simulink model "Differential_Jacobian_mapping_Model"  (R2016a)
settings: Solver=FixedStepAuto  SolverMode=SingleTasking  StartTime=0  StopTime=2  FixedStep=0.04  RelTol=1e-3
undefined symbols (not defined in the file): display, Z
libraries: sm_lib x176, nesl_utility x21, simulink x10
(part 1 of 2)
settings Model: Creator=Andrew  LastModifiedBy=wul20

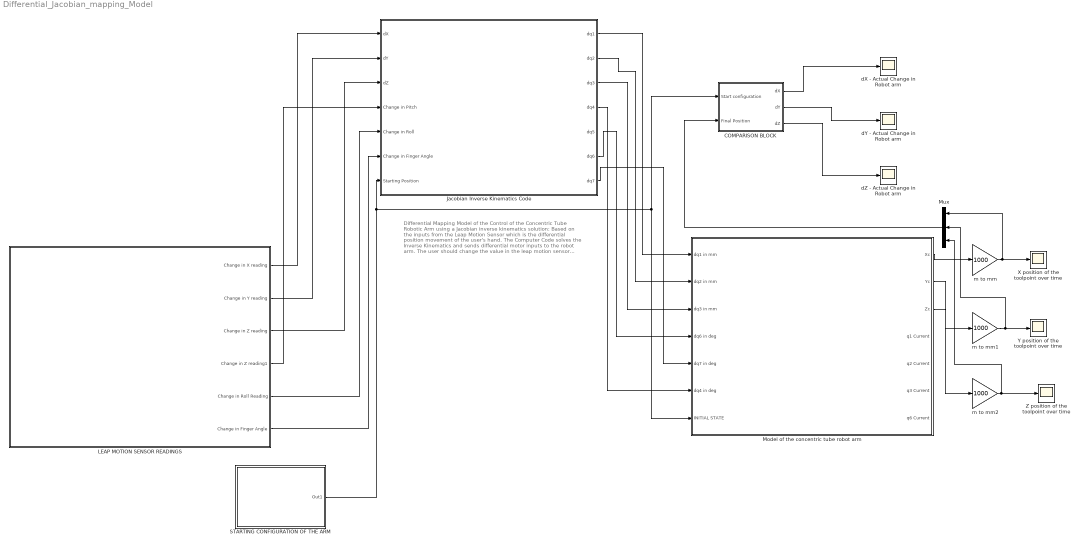
== system Differential_Jacobian_mapping_Model ==
  note: Differential Mapping Model of the Control of
      | the Concentric Tube Robotic Arm using a Jacobian inverse kinematics solution:
      |
      | Based on the inputs from the Leap Motion Sensor which is the differential position movement of the user's hand.
      | The Computer Code solves the Inverse Kinematics and sends differential motor inputs to the robot arm.
      |
      | The user should change the value in the leap motion sensor readings and see how the differential mapping model sends the right motor commands to the arm for it to reach the desired position-change recorded in the scopes from the comparison block.
      |
      | The extrusion takes about 1 simulation second in this simulation every time it elongates to its target position
  COMPARISON BLOCK : Subsystem
  Jacobian Inverse Kinematics Code : Subsystem
      mask Display: image('computer.png');
  LEAP MOTION SENSOR READINGS : Subsystem  mask{X=10, Y=-10, Z=10, P=0, R=90, d=60}
      mask prompts: X "Change in Toolpoint X position (mm)"; Y "Change in Toolpoint Y position (mm)"; Z "Change in Toolpoint Z position (mm)"; P "Change in hand pitch position (degrees)"; R "Change in Roll Angle (degrees)"; d "Change in Finger angle (degrees)"
      mask help: Write down the target differential displacement and orientation:
      mask Display: image('Leap motion Sensor.png');
  Model of the concentric tube robot arm : Subsystem  mask(3D Model of the Concentric Tube Robot Arm){r=173.58}
      mask prompts: r "Radius of curvature in mm"
      mask help:
      | This is a simmechanics model of the robot arm extruding from the origin to its destination in a constant 1 second.
      | Due to the limitations in the model, the maximum extrusion are:
      | tube 1 extrudes a maximum of 100mm (relative)
      | tube 2 extrudes a maximum of 272.67mm that is 90 degrees of curvature (relative)
      | tube 3 extrudes a maximum of 300mm (relative)
      mask init:
      | %set_param('Differential_Jacobian_mapping_Model','AlgebraicLoopSolver','LineSearch')
      | set_param('Differential_Jacobian_mapping_Model','AlgebraicLoopSolver','TrustRegion')
      | 
      | % Geometry 
      | r = 173.58;
      | 
      | %initial Joint conditions:
      | q1 = 10;
      | q2 = 30;
      | q3 = 7;
      | 
      | %Cross section of the Curved Tube
      | x = [-1:0.01:1];
      | y = [sqrt(1-x.^2) -sqrt(1-x.^2)];
      | x = r + x;
      | X = [x'; flip(x)'];
      | Y = y';
      | Cross_section_tube2 = [X, flip(Y)];
      | Cross_section_tube2(202,:)=[];
      | Cross_section_tube2(401,:)=[];
      mask Display: image('Concentric tube robot picture.png');
  Mux : Mux  Inputs=3
  STARTING CONFIGURATION OF THE ARM : Subsystem  mask{q1_in=50, q2_in=50, q3_in=50, q6_in=90, q7_in=0}
      mask prompts: q1_in "Initial q1 elongation (mm)"; q2_in "Initial q2 elongation (mm)"; q3_in "Initial q3 elongation (mm)"; q6_in "Initial q6 rotation (degrees) e.g. 0 degrees means the arm points downwards"; q7_in "Initial q7 rotation (degrees)"
  X position of the toolpoint over time : Scope
  Y position of the toolpoint over time : Scope
  Z position of the toolpoint over time : Scope
  dX - Actual Change in Robot arm : Scope
  dY - Actual Change in Robot arm : Scope
  dZ - Actual Change in Robot arm : Scope
  m to mm : Gain  Gain=1000
  m to mm1 : Gain  Gain=1000
  m to mm2 : Gain  Gain=1000
  wires:
  Model of the concentric tube robot arm/2(Yc) -> m to mm1/1
  Model of the concentric tube robot arm/1(Xc) -> m to mm/1
  Model of the concentric tube robot arm/3(Zc) -> m to mm2/1
  LEAP MOTION SENSOR READINGS/1(Change in X reading) -> Jacobian Inverse Kinematics Code/1(dX)
  LEAP MOTION SENSOR READINGS/2(Change in Y reading) -> Jacobian Inverse Kinematics Code/2(dY)
  LEAP MOTION SENSOR READINGS/3(Change in Z reading) -> Jacobian Inverse Kinematics Code/3(dZ)
  LEAP MOTION SENSOR READINGS/5(Change in Roll Reading) -> Jacobian Inverse Kinematics Code/5(Change in Roll)
  m to mm/1 -> Mux/1, X position of the toolpoint over time/1
  m to mm1/1 -> Mux/2, Y position of the toolpoint over time/1
  m to mm2/1 -> Z position of the toolpoint over time/1, Mux/3
  LEAP MOTION SENSOR READINGS/6(Change in Finger Angle) -> Jacobian Inverse Kinematics Code/6(Change in Finger Angle)
  Jacobian Inverse Kinematics Code/1(dq1) -> Model of the concentric tube robot arm/1(dq1 in mm)
  Jacobian Inverse Kinematics Code/2(dq2) -> Model of the concentric tube robot arm/2(dq2 in mm)
  Jacobian Inverse Kinematics Code/3(dq3) -> Model of the concentric tube robot arm/3(dq3 in mm)
  Jacobian Inverse Kinematics Code/7(dq7) -> Model of the concentric tube robot arm/5(dq7 in deg)
  STARTING CONFIGURATION OF THE ARM/1(Out1) -> Jacobian Inverse Kinematics Code/7(Starting Position), COMPARISON BLOCK/1(Start configuration), Model of the concentric tube robot arm/7(INITIAL STATE)
  Jacobian Inverse Kinematics Code/4(dq4) -> Model of the concentric tube robot arm/6(dq4 in deg)
  Mux/1 -> COMPARISON BLOCK/2(Final Position)
  COMPARISON BLOCK/1(dX) -> dX - Actual Change in Robot arm/1
  COMPARISON BLOCK/2(dY) -> dY - Actual Change in Robot arm/1
  COMPARISON BLOCK/3(dZ) -> dZ - Actual Change in Robot arm/1
  Jacobian Inverse Kinematics Code/6(dq6) -> Model of the concentric tube robot arm/4(dq6 in deg)
  LEAP MOTION SENSOR READINGS/4(Change in Z reading1) -> Jacobian Inverse Kinematics Code/4(Change in Pitch)

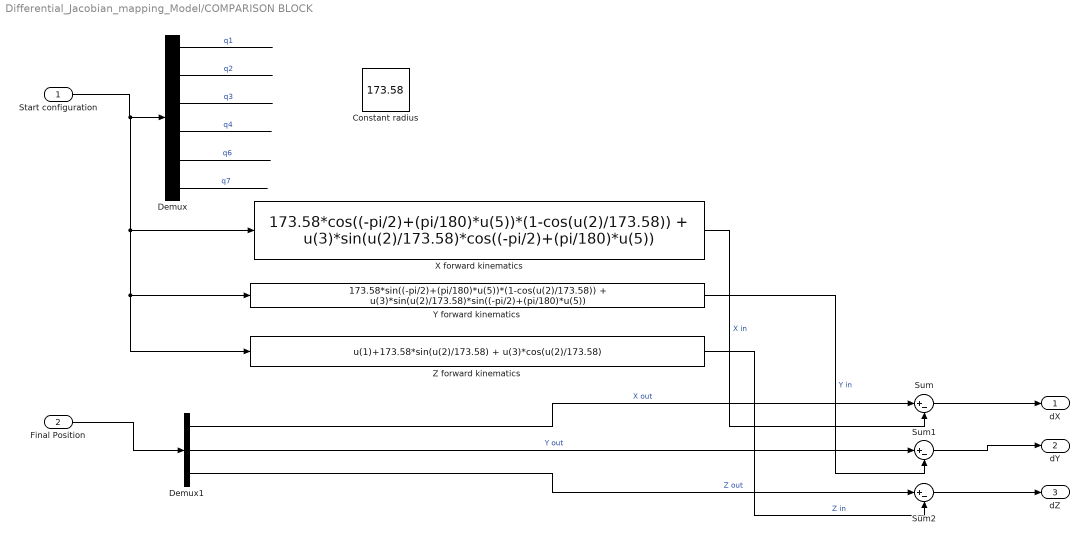
== system Differential_Jacobian_mapping_Model/COMPARISON BLOCK ==
  Start configuration : Inport
  Final Position : Inport  Port=2
  Constant radius : Constant  Value=173.58
  Demux : Demux  Outputs=6
  Demux1 : Demux  Outputs=3
  Sum : Sum  Inputs=|+-
  Sum1 : Sum  Inputs=|+-
  Sum2 : Sum  Inputs=|+-
  X forward kinematics : Fcn  Expr=173.58*cos((-pi/2)+(pi/180)*u(5))*(1-cos(u(2)/173.58)) + u(3)*sin(u(2)/173.58)*cos((-pi/2)+(pi/180)*u(5))
  Y forward kinematics : Fcn  Expr=173.58*sin((-pi/2)+(pi/180)*u(5))*(1-cos(u(2)/173.58)) + u(3)*sin(u(2)/173.58)*sin((-pi/2)+(pi/180)*u(5))
  Z forward kinematics : Fcn  Expr=u(1)+173.58*sin(u(2)/173.58) + u(3)*cos(u(2)/173.58)
  dX : Outport
  dY : Outport  Port=2
  dZ : Outport  Port=3
  wires:
  Start configuration/1 -> Z forward kinematics/1, Y forward kinematics/1, X forward kinematics/1, Demux/1
  Demux/1 -> ?  "q1"
  Demux/2 -> ?  "q2"
  Demux/3 -> ?  "q3"
  Demux/4 -> ?  "q4"
  Demux/5 -> ?  "q6"
  Demux/6 -> ?  "q7"
  X forward kinematics/1 -> Sum/2  "X in"
  Y forward kinematics/1 -> Sum1/2  "Y in"
  Z forward kinematics/1 -> Sum2/2  "Z in"
  Final Position/1 -> Demux1/1
  Demux1/1 -> Sum/1  "X out"
  Demux1/2 -> Sum1/1  "Y out"
  Demux1/3 -> Sum2/1  "Z out"
  Sum2/1 -> dZ/1
  Sum1/1 -> dY/1
  Sum/1 -> dX/1

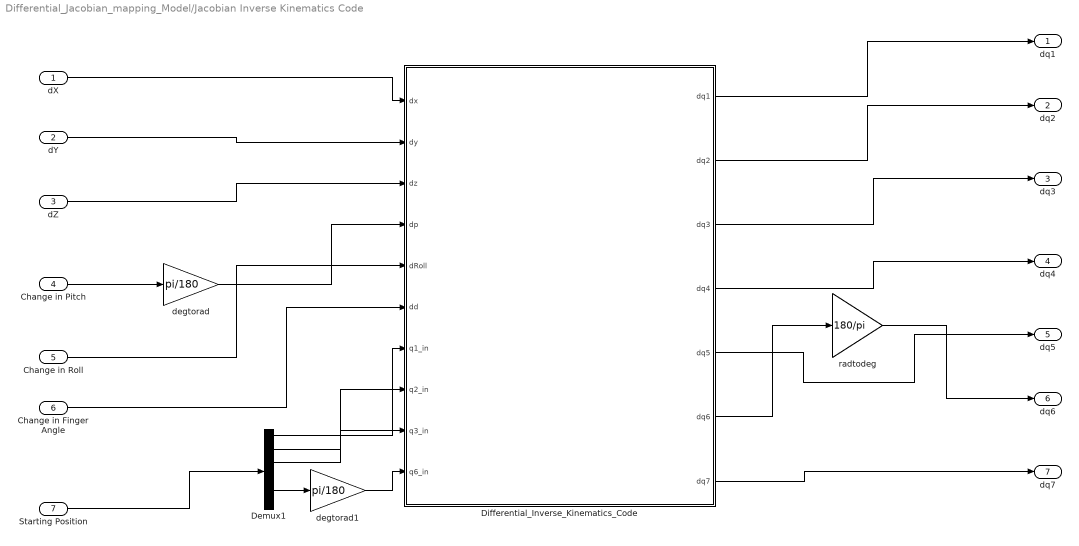
== system Differential_Jacobian_mapping_Model/Jacobian Inverse Kinematics Code ==
  dX : Inport
  dY : Inport  Port=2
  dZ : Inport  Port=3
  Change in Pitch : Inport  Port=4
  Change in Roll : Inport  Port=5
  Change in Finger Angle : Inport  Port=6
  Starting Position : Inport  Port=7
  Demux1 : Demux  Outputs=6
  Differential_Inverse_Kinematics_Code : MATLAB Function  TreatAsAtomicUnit=on
  degtorad : Gain  Gain=pi/180
  degtorad1 : Gain  Gain=pi/180
  radtodeg : Gain  Gain=180/pi
  dq1 : Outport
  dq2 : Outport  Port=2
  dq3 : Outport  Port=3
  dq4 : Outport  Port=4
  dq5 : Outport  Port=5
  dq6 : Outport  Port=6
  dq7 : Outport  Port=7
  wires:
  dX/1 -> Differential_Inverse_Kinematics_Code/1(dx)
  dY/1 -> Differential_Inverse_Kinematics_Code/2(dy)
  dZ/1 -> Differential_Inverse_Kinematics_Code/3(dz)
  Change in Roll/1 -> Differential_Inverse_Kinematics_Code/5(dRoll)
  Differential_Inverse_Kinematics_Code/1(dq1) -> dq1/1
  Differential_Inverse_Kinematics_Code/2(dq2) -> dq2/1
  Differential_Inverse_Kinematics_Code/3(dq3) -> dq3/1
  Differential_Inverse_Kinematics_Code/4(dq4) -> dq4/1
  Differential_Inverse_Kinematics_Code/5(dq5) -> dq5/1
  Differential_Inverse_Kinematics_Code/7(dq7) -> dq7/1
  Change in Pitch/1 -> degtorad/1
  degtorad/1 -> Differential_Inverse_Kinematics_Code/4(dp)
  Differential_Inverse_Kinematics_Code/6(dq6) -> radtodeg/1
  radtodeg/1 -> dq6/1
  Change in Finger Angle/1 -> Differential_Inverse_Kinematics_Code/6(dd)
  Starting Position/1 -> Demux1/1
  Demux1/1 -> Differential_Inverse_Kinematics_Code/7(q1_in)
  Demux1/2 -> Differential_Inverse_Kinematics_Code/8(q2_in)
  Demux1/3 -> Differential_Inverse_Kinematics_Code/9(q3_in)
  degtorad1/1 -> Differential_Inverse_Kinematics_Code/10(q6_in)
  Demux1/5 -> degtorad1/1

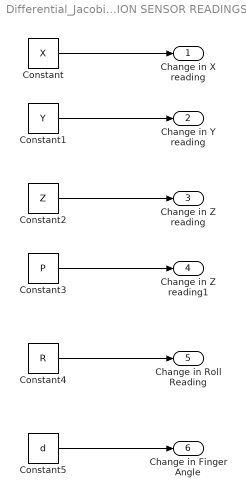
== system Differential_Jacobian_mapping_Model/LEAP MOTION SENSOR READINGS ==
  Constant : Constant  Value=X
  Constant1 : Constant  Value=Y
  Constant2 : Constant  Value=Z
  Constant3 : Constant  Value=P
  Constant4 : Constant  Value=R
  Constant5 : Constant  Value=d
  Change in X reading : Outport
  Change in Y reading : Outport  Port=2
  Change in Z reading : Outport  Port=3
  Change in Z reading1 : Outport  Port=4
  Change in Roll Reading : Outport  Port=5
  Change in Finger Angle : Outport  Port=6
  wires:
  Constant/1 -> Change in X reading/1
  Constant1/1 -> Change in Y reading/1
  Constant2/1 -> Change in Z reading/1
  Constant4/1 -> Change in Roll Reading/1
  Constant5/1 -> Change in Finger Angle/1
  Constant3/1 -> Change in Z reading1/1

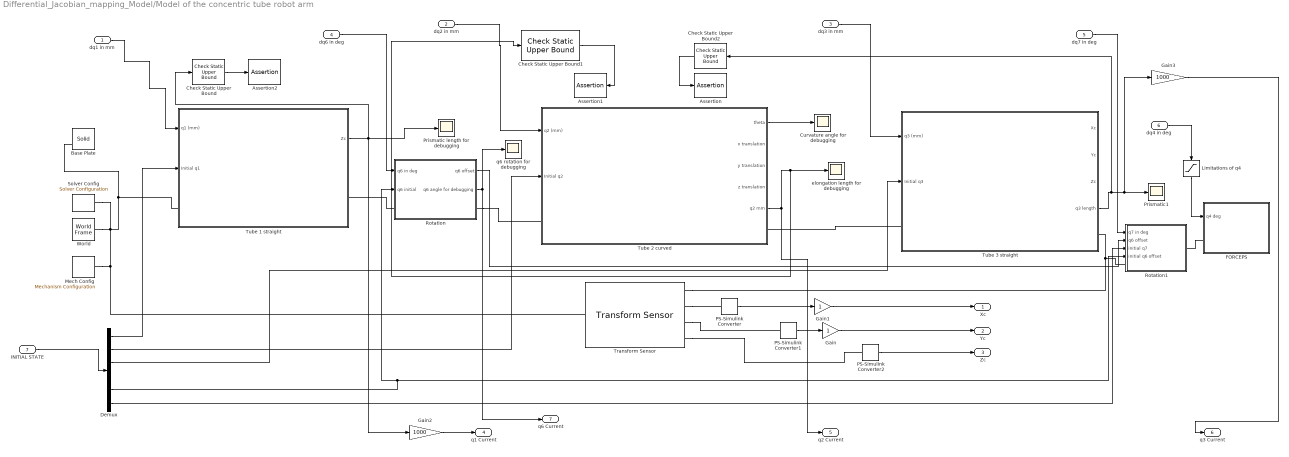
== system Differential_Jacobian_mapping_Model/Model of the concentric tube robot arm ==
  dq1 in mm : Inport
  dq2 in mm : Inport  Port=2
  dq3 in mm : Inport  Port=3
  dq6 in deg : Inport  Port=4
  dq7 in deg : Inport  Port=5
  dq4 in deg : Inport  Port=6
  INITIAL STATE : Inport  Port=7
  Assertion : Assertion  AssertionFailFcn=display('Warning: Tube 3 has reached maximum elongation. You may get an inaccurate position')  StopWhenAssertionFail=off
  Assertion1 : Assertion  AssertionFailFcn=display('Warning: Tube 2 has reached maximum elongation. You may get an inaccurate position')  StopWhenAssertionFail=off
  Assertion2 : Assertion  AssertionFailFcn=display('Warning: Tube 1 has reached maximum elongation. You may get an inaccurate position')  StopWhenAssertionFail=off
  Base Plate : sm_lib/Body Elements/Solid  InertiaType=CalculateFromGeometry  Mass=1  MassUnits=kg  CenterOfMass=[0 0 0]  CenterOfMassUnits=m  MomentsOfInertia=[1 1 1]  MomentsOfInertiaUnits=kg*m^2  ProductsOfInertia=[0 0 0]  ProductsOfInertiaUnits=kg*m^2  DensityBased=on  Density=1000  DensityUnits=kg/(m^3)  DoExposeReferenceFrame=on  SerializedFrames=<Frames><Frame><Id>Frame1</Id><Value><Name>B</Name><Origin><Source>GeometricFeature</Source><FeatureName>+z surface</FeatureName></Origin><PrimaryAxis><DefinedDirection>+Z</DefinedDirection><Source>ReferenceFrame</Source><SourceDirection>+Z</SourceDirection><FeatureName></FeatureName></PrimaryAxis><SecondaryAxis><DefinedDirection>+X</DefinedDirection><Source>ReferenceFrame</Source><SourceDirection>+X</SourceDirection><FeatureName></FeatureName></SecondaryAxis></Value></Frame><Frame><Id>Frame2</Id><Value><Name>F2</Name><Origin><Source>GeometricFeature</Source><FeatureName>+z surface</FeatureName></Origin><PrimaryAxis><DefinedDirection>+Z</DefinedDirection><Source>ReferenceFrame</Source><SourceDirection>+Z</SourceDirection><FeatureName></FeatureName></PrimaryAxis><SecondaryAxis><DefinedDirection>+X</DefinedDirection><Source>ReferenceFrame</Source><SourceDirection>+X</SourceDirection><FeatureName></FeatureName></SecondaryAxis></Value></Frame></Frames>  GraphicType=FromGeometry  MarkerShape=Sphere  MarkerSize=10  GraphicVisPropType=SimpleVisualProperties  GraphicDiffuseColor=[0.4 0.4 0.4]  GraphicSpecularColor=[0.5 0.5 0.5 1.0]  GraphicAmbientColor=[0.15 0.15 0.15 1.0]  GraphicEmissiveColor=[0.0 0.0 0.0 1.0]  GraphicShininess=75  GraphicOpacity=1.0  GeometryShape=Brick  RectangleSize=[1 1]  RectangleSizeUnits=m  BrickDimensions=[100 100 500]  BrickDimensionUnits=mm  CylinderRadius=1  CylinderRadiusUnits=m  CylinderLength=1  CylinderLengthUnits=m  SphereRadius=1  SphereRadiusUnits=m  EllipsoidRadii=[1 1 1]  EllipsoidRadiiUnits=m  ExtrusionCrossSection=10  ExtrusionCrossSectionUnits=cm  ExtrusionLength=10  ExtrusionLengthUnits=cm  PolygonNumSides=3  PolygonOuterRadius=1  PolygonOuterRadiusUnits=m  ExtGeomFileType=STL  ExtGeomFileUnits=m  RevolutionCrossSection=[1 1; 1 -1; 2 -1; 2 1]  RevolutionCrossSectionUnits=m  RevolutionExtent=Full  RevolutionAngle=180  RevolutionAngleUnits=deg
  Check Static Upper Bound : simulink/Model Verification/Check Static  Upper Bound  Description=u <= 0.07725  max=0.07725  max_included=on  enabled=off  callback=Warning: Tube 1 has reached maximum elongation. You may get inaccurate position  stopWhenAssertionFail=off  export=on  icon=text
  Check Static Upper Bound1 : simulink/Model Verification/Check Static  Upper Bound  Description=u <= 82.5  max=82.5  max_included=on  enabled=off  callback=Warning: Tube 2 has reached maximum elongation. You may get inaccurate position  stopWhenAssertionFail=off  export=on  icon=graphic
  Check Static Upper Bound2 : simulink/Model Verification/Check Static  Upper Bound  Description=u <= 0.0975  max=0.0975  max_included=on  enabled=off  callback="\"Warning: Tube 3 has reached maximum elongation. You may get an inaccurate position\""  stopWhenAssertionFail=off  export=on  icon=text
      settings: AttributesFormatString=%<callback>
  Curvature angle for debugging : Scope
  Demux : Demux  Outputs=6
  FORCEPS : Subsystem
      mask Display: image('Forceps.png');
  Gain : Gain
  Gain1 : Gain
  Gain2 : Gain  Gain=1000
  Gain3 : Gain  Gain=1000
  Limitations of q4 : Saturate  UpperLimit=60  LowerLimit=0
  Mech Config : sm_lib/Utilities/Mechanism Configuration  UniformGravity=Constant  GravityVector=[0 0 -9.80665]  GravityUnits=m/s^2  LinearizationDelta=0.001
  PS-Simulink Converter : nesl_utility/PS-Simulink Converter  PhysicalDomain=network_engine_domain  SubClassName=ps_output  LeftPortType=input  RightPortType=output  PseudoPeriodic=off  Frequencies=[]  Unit=1  AffineConversion=off
  PS-Simulink Converter1 : nesl_utility/PS-Simulink Converter  PhysicalDomain=network_engine_domain  SubClassName=ps_output  LeftPortType=input  RightPortType=output  PseudoPeriodic=off  Frequencies=[]  Unit=1  AffineConversion=off
  PS-Simulink Converter2 : nesl_utility/PS-Simulink Converter  PhysicalDomain=network_engine_domain  SubClassName=ps_output  LeftPortType=input  RightPortType=output  PseudoPeriodic=off  Frequencies=[]  Unit=1  AffineConversion=off
  Prismatic length for debugging : Scope
  Prismatic1 : Scope
  Rotation : Subsystem
  Rotation1 : Subsystem
  Solver Config : nesl_utility/Solver Configuration  PhysicalDomain=network_engine_domain  SubClassName=solver  LeftPortType=input  RightPortType=generic  Accelerate=off  Tones=[]  Harmonics=[]  SimulateNoise=off  Profile=off  UseLocalSampling=off  EnableSwitchedLinearOptims=on  FrequencyDomain=off  UseCCode=off  RelTol=0.001  AbsTol=1e-06  MinStep=1e-09  ToWorkspace=off  RevertToSquareIcSolve=off  NumHomotopyIterations=100  PhasorMode=off  PhasorModeNumHarmonics=1  OverrideAbsTol=off  DoDC=off  ResidualTolerance=1e-06  UseLocalSolver=off  LocalSolverChoice=NE_BACKWARD_EULER_ADVANCER  LocalSolverSampleTime=0.001  DoFixedCost=off  MaxNonlinIter=3  MaxModeIter=2  LinearAlgebra=Sparse  DelaysMemoryBudget=1024  AutomaticFiltering=on  FilteringTimeConstant=0.001
  Transform Sensor : sm_lib/Frames and Transforms/Transform Sensor  MeasurementFrame=Base  SenseAngle=off  SenseAxis=off  SenseAngle1=off  SenseAngle2=off  SenseAngle3=off  SenseQ=off  SenseR=off  SenseOmegaX=off  SenseOmegaY=off  SenseOmegaZ=off  SenseOmega1=off  SenseOmega2=off  SenseOmega3=off  SenseQDot=off  SenseRDot=off  SenseAlphaX=off  SenseAlphaY=off  SenseAlphaZ=off  SenseAlpha1=off  SenseAlpha2=off  SenseAlpha3=off  SenseQDDot=off  SenseRDDot=off  SenseX=on  SenseY=on  SenseZ=on  SenseRad=off  SenseAzim=off  SenseDist=off  SenseInc=off  SenseXDot=off  SenseYDot=off  SenseZDot=off  SenseRadDot=off  SenseAzimDot=off  SenseDistDot=off  SenseIncDot=off  SenseXDDot=off  SenseYDDot=off  SenseZDDot=off  SenseRadDDot=off  SenseAzimDDot=off  SenseDistDDot=off  SenseIncDDot=off
  Tube 1 straight : Subsystem
      mask Display: image('straight tube.png');
  Tube 2 curved : Subsystem
      mask Display: image('The curved tube.png');
  Tube 3 straight : Subsystem
      mask Display: image('straight tube.png');
  World : sm_lib/Frames and Transforms/World Frame
  elongation length for debugging : Scope
  q6 rotation for debugging : Scope
  Xc : Outport
  Yc : Outport  Port=2
  Zc : Outport  Port=3
  q1 Current : Outport  Port=4
  q2 Current : Outport  Port=5
  q3 Current : Outport  Port=6
  q6 Current : Outport  Port=7
  wires:
  dq1 in mm/1 -> Tube 1 straight/1(q1 (mm))
  dq2 in mm/1 -> Tube 2 curved/1(q2 (mm))
  dq3 in mm/1 -> Tube 3 straight/1(q3 (mm))
  PS-Simulink Converter1/1 -> Gain/1
  PS-Simulink Converter2/1 -> Zc/1
  PS-Simulink Converter/1 -> Gain1/1
  Gain/1 -> Yc/1
  dq6 in deg/1 -> Rotation/1(q6 in deg)
  dq7 in deg/1 -> Rotation1/1(q7 in deg)
  dq4 in deg/1 -> Limitations of q4/1
  Limitations of q4/1 -> FORCEPS/1(q4 deg)
  Tube 1 straight/1(Zc) -> Gain2/1, Check Static Upper Bound/1, Prismatic length for debugging/1
  Tube 2 curved/1(theta) -> Curvature angle for debugging/1
  Rotation/1(q6 offset) -> Rotation1/2(q6 offset)
  Check Static Upper Bound2/1 -> Assertion/1
  Check Static Upper Bound1/1 -> Assertion1/1
  Check Static Upper Bound/1 -> Assertion2/1
  Gain1/1 -> Xc/1
  INITIAL STATE/1 -> Demux/1
  Demux/1 -> Tube 1 straight/2(Initial q1)
  Demux/5 -> Rotation1/4(initial q6 offset), Rotation/2(q6 initial)
  Demux/2 -> Tube 2 curved/2(Initial q2)
  Demux/3 -> Tube 3 straight/2(Initial q3)
  Demux/6 -> Rotation1/3(initial q7)
  Rotation/2(q6 angle for debugging) -> q6 rotation for debugging/1, q6 Current/1
  Tube 3 straight/4(q3 length) -> Check Static Upper Bound2/1, Gain3/1, Prismatic1/1
  Tube 2 curved/5(q2 mm) -> Check Static Upper Bound1/1, elongation length for debugging/1, q2 Current/1
  Gain2/1 -> q1 Current/1
  Gain3/1 -> q3 Current/1
  connections:
  World/RConn1 -- Transform Sensor/LConn1 -- Mech Config/RConn1 -- Tube 1 straight/LConn1 -- Base Plate/LConn2 -- Solver Config/RConn1
  Tube 3 straight/LConn1 -- Tube 2 curved/RConn1
  Transform Sensor/RConn4 -- PS-Simulink Converter2/LConn1
  Transform Sensor/RConn1 -- Tube 3 straight/RConn1 -- Rotation1/LConn1
  Rotation/LConn1 -- Tube 1 straight/RConn1
  Rotation/RConn1 -- Tube 2 curved/LConn1
  FORCEPS/LConn1 -- Rotation1/RConn1
  Transform Sensor/RConn3 -- PS-Simulink Converter1/LConn1
  Transform Sensor/RConn2 -- PS-Simulink Converter/LConn1

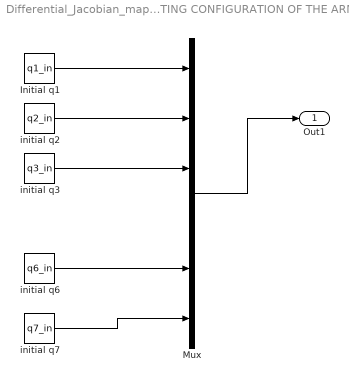
== system Differential_Jacobian_mapping_Model/STARTING CONFIGURATION OF THE ARM ==
  Initial q1 : Constant  Value=q1_in
  Mux : Mux  Inputs=6
  initial q2 : Constant  Value=q2_in
  initial q3 : Constant  Value=q3_in
  initial q6 : Constant  Value=q6_in
  initial q7 : Constant  Value=q7_in
  Out1 : Outport
  wires:
  Mux/1 -> Out1/1
  Initial q1/1 -> Mux/1
  initial q2/1 -> Mux/2
  initial q3/1 -> Mux/3
  initial q6/1 -> Mux/5
  initial q7/1 -> Mux/6

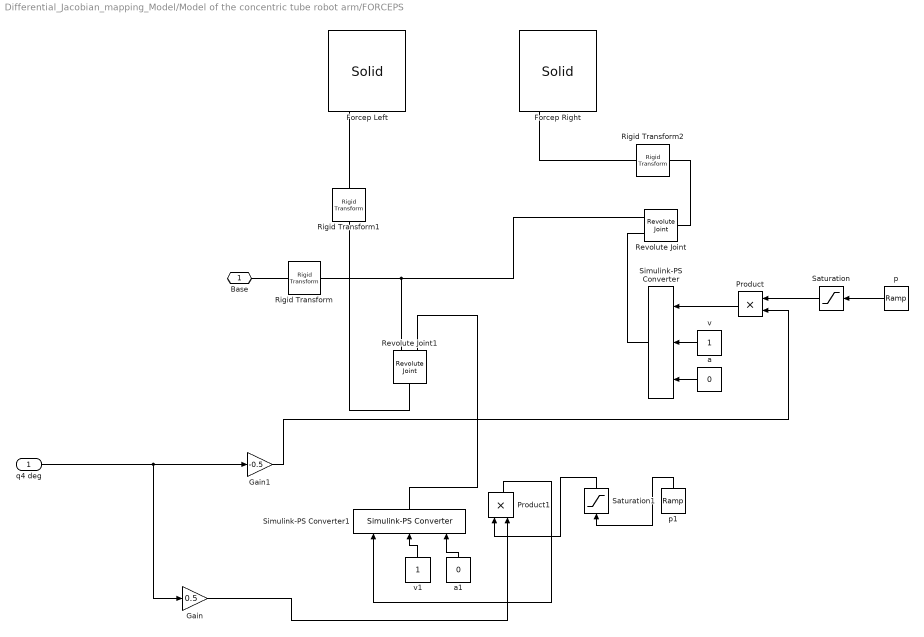
== system Differential_Jacobian_mapping_Model/Model of the concentric tube robot arm/FORCEPS ==
  q4 deg : Inport
  Forcep Left : sm_lib/Body Elements/Solid  InertiaType=CalculateFromGeometry  Mass=1  MassUnits=kg  CenterOfMass=[0 0 0]  CenterOfMassUnits=m  MomentsOfInertia=[1 1 1]  MomentsOfInertiaUnits=kg*m^2  ProductsOfInertia=[0 0 0]  ProductsOfInertiaUnits=kg*m^2  DensityBased=on  Density=1000  DensityUnits=kg/(m^3)  DoExposeReferenceFrame=on  SerializedFrames=<Frames><Frame><Id>Frame1</Id><Value><Name>Rot</Name><Origin><Source>ReferenceFrame</Source><FeatureName></FeatureName></Origin><PrimaryAxis><DefinedDirection>+Z</DefinedDirection><Source>ReferenceFrame</Source><SourceDirection>+Z</SourceDirection><FeatureName></FeatureName></PrimaryAxis><SecondaryAxis><DefinedDirection>+X</DefinedDirection><Source>ReferenceFrame</Source><SourceDirection>+X</SourceDirection><FeatureName></FeatureName></SecondaryAxis></Value></Frame><Frame><Id>Frame2</Id><Value><Name>base</Name><Origin><Source>GeometricFeature</Source><FeatureName>side curve 4</FeatureName></Origin><PrimaryAxis><DefinedDirection>+Y</DefinedDirection><Source>ReferenceFrame</Source><SourceDirection>+Z</SourceDirection><FeatureName></FeatureName></PrimaryAxis><SecondaryAxis><DefinedDirection>+X</DefinedDirection><Source>ReferenceFrame</Source><SourceDirection>+Y</SourceDirection><FeatureName></FeatureName></SecondaryAxis></Value></Frame></Frames>  GraphicType=FromGeometry  MarkerShape=Sphere  MarkerSize=10  GraphicVisPropType=SimpleVisualProperties  GraphicDiffuseColor=[0.5 0.5 0.5]  GraphicSpecularColor=[0.5 0.5 0.5 1.0]  GraphicAmbientColor=[0.15 0.15 0.15 1.0]  GraphicEmissiveColor=[0.0 0.0 0.0 1.0]  GraphicShininess=75  GraphicOpacity=1.0  GeometryShape=GeneralExtrusion  RectangleSize=[1 1]  RectangleSizeUnits=m  BrickDimensions=[1 1 1]  BrickDimensionUnits=m  CylinderRadius=1  CylinderRadiusUnits=m  CylinderLength=1  CylinderLengthUnits=m  SphereRadius=1  SphereRadiusUnits=m  EllipsoidRadii=[1 1 1]  EllipsoidRadiiUnits=m  ExtrusionCrossSection=[3 0; 2 1; 0 1; 0 0]  ExtrusionCrossSectionUnits=mm  ExtrusionLength=1  ExtrusionLengthUnits=mm  PolygonNumSides=3  PolygonOuterRadius=1  PolygonOuterRadiusUnits=m  ExtGeomFileType=STEP  ExtGeomFileUnits=m  RevolutionCrossSection=[1 1; 1 -1; 2 -1; 2 1]  RevolutionCrossSectionUnits=m  RevolutionExtent=Full  RevolutionAngle=180  RevolutionAngleUnits=deg
  Forcep Right : sm_lib/Body Elements/Solid  InertiaType=CalculateFromGeometry  Mass=1  MassUnits=kg  CenterOfMass=[0 0 0]  CenterOfMassUnits=m  MomentsOfInertia=[1 1 1]  MomentsOfInertiaUnits=kg*m^2  ProductsOfInertia=[0 0 0]  ProductsOfInertiaUnits=kg*m^2  DensityBased=on  Density=1000  DensityUnits=kg/(m^3)  DoExposeReferenceFrame=on  SerializedFrames=<Frames><Frame><Id>Frame1</Id><Value><Name>Rot</Name><Origin><Source>ReferenceFrame</Source><FeatureName></FeatureName></Origin><PrimaryAxis><DefinedDirection>+Z</DefinedDirection><Source>ReferenceFrame</Source><SourceDirection>+Z</SourceDirection><FeatureName></FeatureName></PrimaryAxis><SecondaryAxis><DefinedDirection>+X</DefinedDirection><Source>ReferenceFrame</Source><SourceDirection>+X</SourceDirection><FeatureName></FeatureName></SecondaryAxis></Value></Frame><Frame><Id>Frame2</Id><Value><Name>base</Name><Origin><Source>GeometricFeature</Source><FeatureName>side curve 2</FeatureName></Origin><PrimaryAxis><DefinedDirection>+Y</DefinedDirection><Source>ReferenceFrame</Source><SourceDirection>+Z</SourceDirection><FeatureName></FeatureName></PrimaryAxis><SecondaryAxis><DefinedDirection>+X</DefinedDirection><Source>ReferenceFrame</Source><SourceDirection>+Y</SourceDirection><FeatureName></FeatureName></SecondaryAxis></Value></Frame></Frames>  GraphicType=FromGeometry  MarkerShape=Sphere  MarkerSize=10  GraphicVisPropType=SimpleVisualProperties  GraphicDiffuseColor=[0.5 0.5 0.5]  GraphicSpecularColor=[0.5 0.5 0.5 1.0]  GraphicAmbientColor=[0.15 0.15 0.15 1.0]  GraphicEmissiveColor=[0.0 0.0 0.0 1.0]  GraphicShininess=75  GraphicOpacity=1.0  GeometryShape=GeneralExtrusion  RectangleSize=[1 1]  RectangleSizeUnits=m  BrickDimensions=[1 1 1]  BrickDimensionUnits=m  CylinderRadius=1  CylinderRadiusUnits=m  CylinderLength=1  CylinderLengthUnits=m  SphereRadius=1  SphereRadiusUnits=m  EllipsoidRadii=[1 1 1]  EllipsoidRadiiUnits=m  ExtrusionCrossSection=[3 0; 0 0; 0 -1; 2 -1]  ExtrusionCrossSectionUnits=mm  ExtrusionLength=1  ExtrusionLengthUnits=mm  PolygonNumSides=3  PolygonOuterRadius=1  PolygonOuterRadiusUnits=m  ExtGeomFileType=STEP  ExtGeomFileUnits=m  RevolutionCrossSection=[1 1; 1 -1; 2 -1; 2 1]  RevolutionCrossSectionUnits=m  RevolutionExtent=Full  RevolutionAngle=180  RevolutionAngleUnits=deg
  Gain : Gain  Gain=0.5
  Gain1 : Gain  Gain=-0.5
  Product : Product
  Product1 : Product
  Revolute Joint : sm_lib/Joints/Revolute Joint  SenseConstraintForce=off  SenseConstraintForceX=off  SenseConstraintForceY=off  SenseConstraintForceZ=off  SenseConstraintTorque=off  SenseConstraintTorqueX=off  SenseConstraintTorqueY=off  SenseConstraintTorqueZ=off  SenseTotalForce=off  SenseTotalForceX=off  SenseTotalForceY=off  SenseTotalForceZ=off  SenseTotalTorque=off  SenseTotalTorqueX=off  SenseTotalTorqueY=off  SenseTotalTorqueZ=off  CompositeWrenchDir=FollowerOnBase  CompositeWrenchFrame=BaseFrame  EquilibriumPosition=0  EquilibriumPositionUnits=deg  SpringStiffness=0  SpringStiffnessUnits=N*m/deg  DampingCoefficient=0  DampingCoefficientUnits=N*m/(deg/s)  TorqueActuationMode=ComputedTorque  MotionActuationMode=InputMotion  SensePosition=off  SenseVelocity=off  SenseAcceleration=off  SenseTorqueForce=off  PositionTargetSpecify=off  PositionTargetPriority=High  PositionTargetValue=0  PositionTargetValueUnits=deg  VelocityTargetSpecify=off  VelocityTargetPriority=High  VelocityTargetValue=0  VelocityTargetValueUnits=deg/s
  Revolute Joint1 : sm_lib/Joints/Revolute Joint  SenseConstraintForce=off  SenseConstraintForceX=off  SenseConstraintForceY=off  SenseConstraintForceZ=off  SenseConstraintTorque=off  SenseConstraintTorqueX=off  SenseConstraintTorqueY=off  SenseConstraintTorqueZ=off  SenseTotalForce=off  SenseTotalForceX=off  SenseTotalForceY=off  SenseTotalForceZ=off  SenseTotalTorque=off  SenseTotalTorqueX=off  SenseTotalTorqueY=off  SenseTotalTorqueZ=off  CompositeWrenchDir=FollowerOnBase  CompositeWrenchFrame=BaseFrame  EquilibriumPosition=0  EquilibriumPositionUnits=deg  SpringStiffness=0  SpringStiffnessUnits=N*m/deg  DampingCoefficient=0  DampingCoefficientUnits=N*m/(deg/s)  TorqueActuationMode=ComputedTorque  MotionActuationMode=InputMotion  SensePosition=off  SenseVelocity=off  SenseAcceleration=off  SenseTorqueForce=off  PositionTargetSpecify=off  PositionTargetPriority=High  PositionTargetValue=0  PositionTargetValueUnits=deg  VelocityTargetSpecify=off  VelocityTargetPriority=High  VelocityTargetValue=0  VelocityTargetValueUnits=deg/s
  Rigid Transform : sm_lib/Frames and Transforms/Rigid Transform  TranslationMethod=None  TranslationLengthUnit=m  TranslationStandardAxis=+Z  TranslationStandardOffset=0  TranslationCartesianOffset=[0 0 0]  TranslationROffset=0  TranslationROffsetUnits=m  TranslationZOffset=0  TranslationZOffsetUnits=m  TranslationThetaOffset=0  TranslationThetaOffsetUnits=deg  RotationMethod=StandardAxis  RotationAngleUnits=deg  RotationStandardAxis=+X  RotationAngle=90  RotationArbitraryAxis=[0 0 1]  FollAlignAxisA=+X  BaseAlignAxisA=+Y  FollAlignAxisB=+Y  BaseAlignAxisB=+Z  RotationSequenceAxes=FollowerAxes  RotationSequence=XYX  RotationSequenceAngles=[0 0 0]  RotationSequenceAnglesUnits=deg  RotationMatrix=[1 0 0; 0 1 0; 0 0 1]
  Rigid Transform1 : sm_lib/Frames and Transforms/Rigid Transform  TranslationMethod=None  TranslationLengthUnit=m  TranslationStandardAxis=+Z  TranslationStandardOffset=0  TranslationCartesianOffset=[0 0 0]  TranslationROffset=0  TranslationROffsetUnits=m  TranslationZOffset=0  TranslationZOffsetUnits=m  TranslationThetaOffset=0  TranslationThetaOffsetUnits=deg  RotationMethod=StandardAxis  RotationAngleUnits=deg  RotationStandardAxis=+Z  RotationAngle=90  RotationArbitraryAxis=[0 0 1]  FollAlignAxisA=+X  BaseAlignAxisA=+Y  FollAlignAxisB=+Y  BaseAlignAxisB=+Z  RotationSequenceAxes=FollowerAxes  RotationSequence=XYX  RotationSequenceAngles=[0 0 0]  RotationSequenceAnglesUnits=deg  RotationMatrix=[1 0 0; 0 1 0; 0 0 1]
  Rigid Transform2 : sm_lib/Frames and Transforms/Rigid Transform  TranslationMethod=None  TranslationLengthUnit=m  TranslationStandardAxis=+Z  TranslationStandardOffset=0  TranslationCartesianOffset=[0 0 0]  TranslationROffset=0  TranslationROffsetUnits=m  TranslationZOffset=0  TranslationZOffsetUnits=m  TranslationThetaOffset=0  TranslationThetaOffsetUnits=deg  RotationMethod=StandardAxis  RotationAngleUnits=deg  RotationStandardAxis=+Z  RotationAngle=90  RotationArbitraryAxis=[0 0 1]  FollAlignAxisA=+X  BaseAlignAxisA=+Y  FollAlignAxisB=+Y  BaseAlignAxisB=+Z  RotationSequenceAxes=FollowerAxes  RotationSequence=XYX  RotationSequenceAngles=[0 0 0]  RotationSequenceAnglesUnits=deg  RotationMatrix=[1 0 0; 0 1 0; 0 0 1]
  Saturation : Saturate  UpperLimit=1  LowerLimit=0
  Saturation1 : Saturate  UpperLimit=1  LowerLimit=0
  Simulink-PS Converter : nesl_utility/Simulink-PS Converter  PhysicalDomain=network_engine_domain  SubClassName=ps_input  LeftPortType=input  RightPortType=output  PseudoPeriodic=off  Frequencies=[]  NoiseDistribution=none  NoiseParameters=[]  Unit=deg  AffineConversion=off  InputFiltering=derivs  SimscapeFilterOrder=1  InputFilterTimeConstant=0.001  UdotUserProvided=2
  Simulink-PS Converter1 : nesl_utility/Simulink-PS Converter  PhysicalDomain=network_engine_domain  SubClassName=ps_input  LeftPortType=input  RightPortType=output  PseudoPeriodic=off  Frequencies=[]  NoiseDistribution=none  NoiseParameters=[]  Unit=deg  AffineConversion=off  InputFiltering=derivs  SimscapeFilterOrder=1  InputFilterTimeConstant=0.001  UdotUserProvided=2
  a : Constant  Value=0
  a1 : Constant  Value=0
  p : simulink/Sources/Ramp  slope=1  start=0  X0=0
  p1 : simulink/Sources/Ramp  slope=1  start=0  X0=0
  v : Constant
  v1 : Constant
  Base : PMIOPort  Port=1  Side=Left
  wires:
  a/1 -> Simulink-PS Converter/3
  v/1 -> Simulink-PS Converter/2
  Saturation/1 -> Product/1
  p/1 -> Saturation/1
  a1/1 -> Simulink-PS Converter1/3
  v1/1 -> Simulink-PS Converter1/2
  Saturation1/1 -> Product1/1
  p1/1 -> Saturation1/1
  Gain/1 -> Product1/2
  Gain1/1 -> Product/2
  Product/1 -> Simulink-PS Converter/1
  q4 deg/1 -> Gain/1, Gain1/1
  Product1/1 -> Simulink-PS Converter1/1
  connections:
  Revolute Joint/LConn2 -- Simulink-PS Converter/RConn1
  Revolute Joint/LConn1 -- Rigid Transform/RConn1 -- Revolute Joint1/LConn1
  Revolute Joint1/LConn2 -- Simulink-PS Converter1/RConn1
  Rigid Transform/LConn1 -- Base/RConn1
  Revolute Joint1/RConn1 -- Rigid Transform1/LConn1
  Rigid Transform2/LConn1 -- Revolute Joint/RConn1
  Rigid Transform1/RConn1 -- Forcep Left/LConn1
  Forcep Right/LConn1 -- Rigid Transform2/RConn1

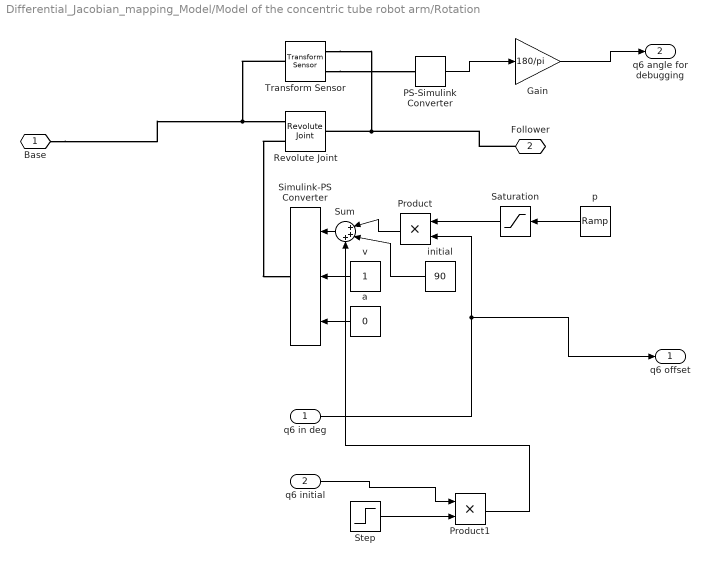
== system Differential_Jacobian_mapping_Model/Model of the concentric tube robot arm/Rotation ==
  q6 in deg : Inport
  q6 initial : Inport  Port=2
  Gain : Gain  Gain=180/pi
  PS-Simulink Converter : nesl_utility/PS-Simulink Converter  PhysicalDomain=network_engine_domain  SubClassName=ps_output  LeftPortType=input  RightPortType=output  PseudoPeriodic=off  Frequencies=[]  Unit=1  AffineConversion=off
  Product : Product
  Product1 : Product
  Revolute Joint : sm_lib/Joints/Revolute Joint  SenseConstraintForce=off  SenseConstraintForceX=off  SenseConstraintForceY=off  SenseConstraintForceZ=off  SenseConstraintTorque=off  SenseConstraintTorqueX=off  SenseConstraintTorqueY=off  SenseConstraintTorqueZ=off  SenseTotalForce=off  SenseTotalForceX=off  SenseTotalForceY=off  SenseTotalForceZ=off  SenseTotalTorque=off  SenseTotalTorqueX=off  SenseTotalTorqueY=off  SenseTotalTorqueZ=off  CompositeWrenchDir=FollowerOnBase  CompositeWrenchFrame=BaseFrame  EquilibriumPosition=0  EquilibriumPositionUnits=deg  SpringStiffness=0  SpringStiffnessUnits=N*m/deg  DampingCoefficient=0  DampingCoefficientUnits=N*m/(deg/s)  TorqueActuationMode=ComputedTorque  MotionActuationMode=InputMotion  SensePosition=off  SenseVelocity=off  SenseAcceleration=off  SenseTorqueForce=off  PositionTargetSpecify=off  PositionTargetPriority=High  PositionTargetValue=0  PositionTargetValueUnits=deg  VelocityTargetSpecify=off  VelocityTargetPriority=High  VelocityTargetValue=0  VelocityTargetValueUnits=deg/s
  Saturation : Saturate  UpperLimit=1  LowerLimit=0
  Simulink-PS Converter : nesl_utility/Simulink-PS Converter  PhysicalDomain=network_engine_domain  SubClassName=ps_input  LeftPortType=input  RightPortType=output  PseudoPeriodic=off  Frequencies=[]  NoiseDistribution=none  NoiseParameters=[]  Unit=deg  AffineConversion=off  InputFiltering=derivs  SimscapeFilterOrder=1  InputFilterTimeConstant=0.001  UdotUserProvided=2
  Step : Step  Time=0  SampleTime=0
  Sum : Sum  Inputs=|+++
  Transform Sensor : sm_lib/Frames and Transforms/Transform Sensor  MeasurementFrame=World  SenseAngle=on  SenseAxis=off  SenseAngle1=off  SenseAngle2=off  SenseAngle3=off  SenseQ=off  SenseR=off  SenseOmegaX=off  SenseOmegaY=off  SenseOmegaZ=off  SenseOmega1=off  SenseOmega2=off  SenseOmega3=off  SenseQDot=off  SenseRDot=off  SenseAlphaX=off  SenseAlphaY=off  SenseAlphaZ=off  SenseAlpha1=off  SenseAlpha2=off  SenseAlpha3=off  SenseQDDot=off  SenseRDDot=off  SenseX=off  SenseY=off  SenseZ=off  SenseRad=off  SenseAzim=off  SenseDist=off  SenseInc=off  SenseXDot=off  SenseYDot=off  SenseZDot=off  SenseRadDot=off  SenseAzimDot=off  SenseDistDot=off  SenseIncDot=off  SenseXDDot=off  SenseYDDot=off  SenseZDDot=off  SenseRadDDot=off  SenseAzimDDot=off  SenseDistDDot=off  SenseIncDDot=off
  a : Constant  Value=0
  initial : Constant  Value=90
  p : simulink/Sources/Ramp  slope=1  start=0  X0=0
  v : Constant
  Base : PMIOPort  Port=1  Side=Left
  Follower : PMIOPort  Port=2  Side=Right
  q6 offset : Outport
  q6 angle for debugging : Outport  Port=2
  wires:
  a/1 -> Simulink-PS Converter/3
  v/1 -> Simulink-PS Converter/2
  Saturation/1 -> Product/1
  p/1 -> Saturation/1
  Sum/1 -> Simulink-PS Converter/1
  initial/1 -> Sum/2
  q6 initial/1 -> Product1/1
  Step/1 -> Product1/2
  Product1/1 -> Sum/3
  PS-Simulink Converter/1 -> Gain/1
  Gain/1 -> q6 angle for debugging/1
  q6 in deg/1 -> Product/2, q6 offset/1
  Product/1 -> Sum/1
  connections:
  Revolute Joint/LConn2 -- Simulink-PS Converter/RConn1
  Base/RConn1 -- Transform Sensor/LConn1 -- Revolute Joint/LConn1
  Follower/RConn1 -- Transform Sensor/RConn1 -- Revolute Joint/RConn1
  Transform Sensor/RConn2 -- PS-Simulink Converter/LConn1

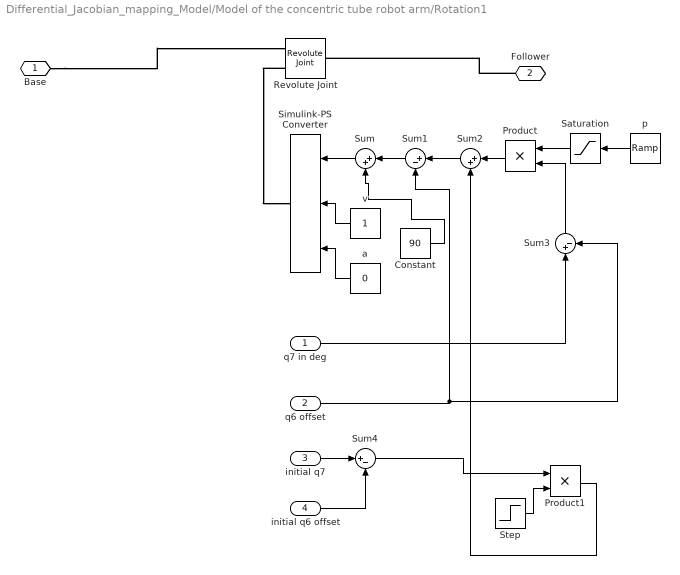
== system Differential_Jacobian_mapping_Model/Model of the concentric tube robot arm/Rotation1 ==
  q7 in deg : Inport
  q6 offset : Inport  Port=2
  initial q7 : Inport  Port=3
  initial q6 offset : Inport  Port=4
  Constant : Constant  Value=90
  Product : Product
  Product1 : Product
  Revolute Joint : sm_lib/Joints/Revolute Joint  SenseConstraintForce=off  SenseConstraintForceX=off  SenseConstraintForceY=off  SenseConstraintForceZ=off  SenseConstraintTorque=off  SenseConstraintTorqueX=off  SenseConstraintTorqueY=off  SenseConstraintTorqueZ=off  SenseTotalForce=off  SenseTotalForceX=off  SenseTotalForceY=off  SenseTotalForceZ=off  SenseTotalTorque=off  SenseTotalTorqueX=off  SenseTotalTorqueY=off  SenseTotalTorqueZ=off  CompositeWrenchDir=FollowerOnBase  CompositeWrenchFrame=BaseFrame  EquilibriumPosition=0  EquilibriumPositionUnits=deg  SpringStiffness=0  SpringStiffnessUnits=N*m/deg  DampingCoefficient=0  DampingCoefficientUnits=N*m/(deg/s)  TorqueActuationMode=ComputedTorque  MotionActuationMode=InputMotion  SensePosition=off  SenseVelocity=off  SenseAcceleration=off  SenseTorqueForce=off  PositionTargetSpecify=off  PositionTargetPriority=High  PositionTargetValue=0  PositionTargetValueUnits=deg  VelocityTargetSpecify=off  VelocityTargetPriority=High  VelocityTargetValue=0  VelocityTargetValueUnits=deg/s
  Saturation : Saturate  UpperLimit=1  LowerLimit=0
  Simulink-PS Converter : nesl_utility/Simulink-PS Converter  PhysicalDomain=network_engine_domain  SubClassName=ps_input  LeftPortType=input  RightPortType=output  PseudoPeriodic=off  Frequencies=[]  NoiseDistribution=none  NoiseParameters=[]  Unit=deg  AffineConversion=off  InputFiltering=derivs  SimscapeFilterOrder=1  InputFilterTimeConstant=0.001  UdotUserProvided=2
  Step : Step  Time=0  SampleTime=0
  Sum : Sum  Inputs=|++
  Sum1 : Sum  Inputs=|+-
  Sum2 : Sum  Inputs=|++
  Sum3 : Sum  Inputs=|+-
  Sum4 : Sum  Inputs=|+-
  a : Constant  Value=0
  p : simulink/Sources/Ramp  slope=1  start=0  X0=0
  v : Constant
  Base : PMIOPort  Port=1  Side=Left
  Follower : PMIOPort  Port=2  Side=Right
  wires:
  a/1 -> Simulink-PS Converter/3
  v/1 -> Simulink-PS Converter/2
  Saturation/1 -> Product/1
  p/1 -> Saturation/1
  Sum/1 -> Simulink-PS Converter/1
  Sum1/1 -> Sum/1
  Step/1 -> Product1/2
  Sum2/1 -> Sum1/1
  q7 in deg/1 -> Sum3/1
  initial q7/1 -> Sum4/1
  Sum4/1 -> Product1/1
  Constant/1 -> Sum/2
  initial q6 offset/1 -> Sum4/2
  Product1/1 -> Sum2/2
  Product/1 -> Sum2/1
  Sum3/1 -> Product/2
  q6 offset/1 -> Sum3/2, Sum1/2
  connections:
  Revolute Joint/LConn2 -- Simulink-PS Converter/RConn1
  Base/RConn1 -- Revolute Joint/LConn1
  Follower/RConn1 -- Revolute Joint/RConn1

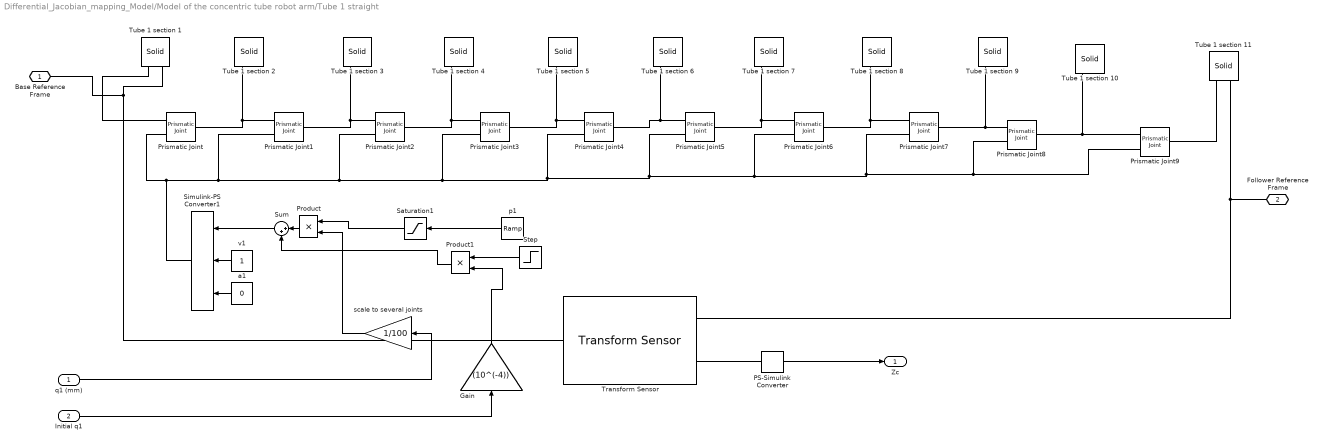
== system Differential_Jacobian_mapping_Model/Model of the concentric tube robot arm/Tube 1 straight ==
  q1 (mm) : Inport
  Initial q1 : Inport  Port=2
  Gain : Gain  Gain=(10^(-4))
  PS-Simulink Converter : nesl_utility/PS-Simulink Converter  PhysicalDomain=network_engine_domain  SubClassName=ps_output  LeftPortType=input  RightPortType=output  PseudoPeriodic=off  Frequencies=[]  Unit=1  AffineConversion=off
  Prismatic Joint{,1..9} (10 alike) : sm_lib/Joints/Prismatic Joint  SenseConstraintForce=off  SenseConstraintForceX=off  SenseConstraintForceY=off  SenseConstraintForceZ=off  SenseConstraintTorque=off  SenseConstraintTorqueX=off  SenseConstraintTorqueY=off  SenseConstraintTorqueZ=off  SenseTotalForce=off  SenseTotalForceX=off  SenseTotalForceY=off  SenseTotalForceZ=off  SenseTotalTorque=off  SenseTotalTorqueX=off  SenseTotalTorqueY=off  SenseTotalTorqueZ=off  CompositeWrenchDir=FollowerOnBase  CompositeWrenchFrame=BaseFrame  EquilibriumPosition=0  EquilibriumPositionUnits=m  SpringStiffness=0  SpringStiffnessUnits=N/m  DampingCoefficient=0  DampingCoefficientUnits=N/(m/s)  TorqueActuationMode=ComputedTorque  MotionActuationMode=InputMotion  SensePosition=off  SenseVelocity=off  SenseAcceleration=off  SenseTorqueForce=off  PositionTargetSpecify=off  PositionTargetPriority=High  PositionTargetValue=0  PositionTargetValueUnits=m  VelocityTargetSpecify=off  VelocityTargetPriority=High  VelocityTargetValue=0  VelocityTargetValueUnits=m/s
  Product : Product
  Product1 : Product
  Saturation1 : Saturate  UpperLimit=0.01  LowerLimit=0
  Simulink-PS Converter1 : nesl_utility/Simulink-PS Converter  PhysicalDomain=network_engine_domain  SubClassName=ps_input  LeftPortType=input  RightPortType=output  PseudoPeriodic=off  Frequencies=[]  NoiseDistribution=none  NoiseParameters=[]  Unit=m  AffineConversion=off  InputFiltering=derivs  SimscapeFilterOrder=1  InputFilterTimeConstant=0.001  UdotUserProvided=2
  Step : Step  Time=0  SampleTime=0
  Sum : Sum  Inputs=|++
  Transform Sensor : sm_lib/Frames and Transforms/Transform Sensor  MeasurementFrame=Base  SenseAngle=off  SenseAxis=off  SenseAngle1=off  SenseAngle2=off  SenseAngle3=off  SenseQ=off  SenseR=off  SenseOmegaX=off  SenseOmegaY=off  SenseOmegaZ=off  SenseOmega1=off  SenseOmega2=off  SenseOmega3=off  SenseQDot=off  SenseRDot=off  SenseAlphaX=off  SenseAlphaY=off  SenseAlphaZ=off  SenseAlpha1=off  SenseAlpha2=off  SenseAlpha3=off  SenseQDDot=off  SenseRDDot=off  SenseX=off  SenseY=off  SenseZ=on  SenseRad=off  SenseAzim=off  SenseDist=off  SenseInc=off  SenseXDot=off  SenseYDot=off  SenseZDot=off  SenseRadDot=off  SenseAzimDot=off  SenseDistDot=off  SenseIncDot=off  SenseXDDot=off  SenseYDDot=off  SenseZDDot=off  SenseRadDDot=off  SenseAzimDDot=off  SenseDistDDot=off  SenseIncDDot=off
  Tube 1 section {1..11} (11 alike) : sm_lib/Body Elements/Solid  InertiaType=CalculateFromGeometry  Mass=1  MassUnits=kg  CenterOfMass=[0 0 0]  CenterOfMassUnits=m  MomentsOfInertia=[1 1 1]  MomentsOfInertiaUnits=kg*m^2  ProductsOfInertia=[0 0 0]  ProductsOfInertiaUnits=kg*m^2  DensityBased=on  Density=0  DensityUnits=kg/(m^3)  DoExposeReferenceFrame=on  SerializedFrames=<Frames><Frame><Id>Frame1</Id><Value><Name>F1</Name><Origin><Source>GeometricFeature</Source><FeatureName>bottom surface</FeatureName></Origin><PrimaryAxis><DefinedDirection>+Z</DefinedDirection><Source>ReferenceFrame</Source><SourceDirection>+Z</SourceDirection><FeatureName></FeatureName></PrimaryAxis><SecondaryAxis><DefinedDirection>+X</DefinedDirection><Source>ReferenceFrame</Source><SourceDirection>+X</SourceDirection><FeatureName></FeatureName></SecondaryAxis></Value></Frame><Frame><Id>Frame2</Id><Value><Name>F2</Name><Origin><Source>GeometricFeature</Source><FeatureName>top surface</FeatureName></Origin><PrimaryAxis><DefinedDirection>+Z</DefinedDirection><Source>ReferenceFrame</Source><SourceDirection>+Z</SourceDirection><FeatureName></FeatureName></PrimaryAxis><SecondaryAxis><DefinedDirection>+X</DefinedDirection><Source>ReferenceFrame</Source><SourceDirection>+X</SourceDirection><FeatureName></FeatureName></SecondaryAxis></Value></Frame></Frames>  GraphicType=FromGeometry  MarkerShape=Sphere  MarkerSize=10  GraphicVisPropType=SimpleVisualProperties  GraphicDiffuseColor=[0.5 0.5 0.5]  GraphicSpecularColor=[0.5 0.5 0.5 1.0]  GraphicAmbientColor=[0.15 0.15 0.15 1.0]  GraphicEmissiveColor=[0.0 0.0 0.0 1.0]  GraphicShininess=75  GraphicOpacity=1.0  GeometryShape=Cylinder  RectangleSize=[1 1]  RectangleSizeUnits=m  BrickDimensions=[1 1 1]  BrickDimensionUnits=m  CylinderRadius=1.5  CylinderRadiusUnits=mm  CylinderLength=10  CylinderLengthUnits=mm  SphereRadius=1  SphereRadiusUnits=m  EllipsoidRadii=[1 1 1]  EllipsoidRadiiUnits=m  ExtrusionCrossSection=[1 1; -1 1; -1 -1; 1 -1]  ExtrusionCrossSectionUnits=m  ExtrusionLength=1  ExtrusionLengthUnits=m  PolygonNumSides=3  PolygonOuterRadius=1  PolygonOuterRadiusUnits=m  ExtGeomFileType=STEP  ExtGeomFileUnits=m  RevolutionCrossSection=[1 1; 1 -1; 2 -1; 2 1]  RevolutionCrossSectionUnits=m  RevolutionExtent=Full  RevolutionAngle=180  RevolutionAngleUnits=deg
  a1 : Constant  Value=0
  p1 : simulink/Sources/Ramp  slope=0.01  start=0  X0=0
  scale to several joints : Gain  Gain=1/100
  v1 : Constant
  Base Reference Frame : PMIOPort  Port=1  Side=Left
  Follower Reference Frame : PMIOPort  Port=2  Side=Right
  Zc : Outport
  wires:
  a1/1 -> Simulink-PS Converter1/3
  v1/1 -> Simulink-PS Converter1/2
  p1/1 -> Saturation1/1
  Saturation1/1 -> Product/1
  PS-Simulink Converter/1 -> Zc/1
  Step/1 -> Product1/1
  Initial q1/1 -> Gain/1
  Product1/1 -> Sum/2
  q1 (mm)/1 -> scale to several joints/1
  Gain/1 -> Product1/2
  scale to several joints/1 -> Product/2
  Product/1 -> Sum/1
  Sum/1 -> Simulink-PS Converter1/1
  connections:
  Prismatic Joint1/LConn2 -- Simulink-PS Converter1/RConn1 -- Prismatic Joint/LConn2 -- Prismatic Joint9/LConn2 -- Prismatic Joint8/LConn2 -- Prismatic Joint7/LConn2 -- Prismatic Joint6/LConn2 -- Prismatic Joint5/LConn2 -- Prismatic Joint4/LConn2 -- Prismatic Joint3/LConn2 -- Prismatic Joint2/LConn2
  Tube 1 section 1/LConn1 -- Prismatic Joint/LConn1
  Prismatic Joint/RConn1 -- Tube 1 section 2/LConn1 -- Prismatic Joint1/LConn1
  Prismatic Joint1/RConn1 -- Tube 1 section 3/LConn1 -- Prismatic Joint2/LConn1
  Tube 1 section 4/LConn1 -- Prismatic Joint2/RConn1 -- Prismatic Joint3/LConn1
  Tube 1 section 5/LConn1 -- Prismatic Joint3/RConn1 -- Prismatic Joint4/LConn1
  Tube 1 section 6/LConn1 -- Prismatic Joint5/LConn1 -- Prismatic Joint4/RConn1
  Prismatic Joint5/RConn1 -- Tube 1 section 7/LConn1 -- Prismatic Joint6/LConn1
  Prismatic Joint6/RConn1 -- Tube 1 section 8/LConn1 -- Prismatic Joint7/LConn1
  Prismatic Joint7/RConn1 -- Tube 1 section 9/LConn1 -- Prismatic Joint8/LConn1
  Tube 1 section 10/LConn1 -- Prismatic Joint8/RConn1 -- Prismatic Joint9/LConn1
  Prismatic Joint9/RConn1 -- Tube 1 section 11/LConn1
  Transform Sensor/LConn1 -- Base Reference Frame/RConn1 -- Tube 1 section 1/LConn2
  Tube 1 section 11/LConn2 -- Transform Sensor/RConn1 -- Follower Reference Frame/RConn1
  PS-Simulink Converter/LConn1 -- Transform Sensor/RConn2
